simulink library "syntheticFlowGenerator"  (R2020a)
settings: Solver=VariableStepAuto  StartTime=0.0  StopTime=10.0  RelTol=1e-3
libraries: simulink x1
settings Model: Creator=Ayaz  LastModifiedBy=Ayaz

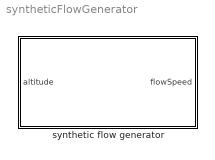
== system syntheticFlowGenerator ==
  synthetic flow generator : Subsystem  mask{hTau='exponential', timeScale=22*60, powerLawParams=[3.77 0.14], tSamp=1*60, finalTime=3*60*60, stdDev=0.5, minFlow=5, rngSeed=1, altScale=200, covAmp=1, zDiscrete=100:100:1000}
      mask prompts: hTau "Temporal kernel"; timeScale "Time scale [s]"; powerLawParams "Power law parameters, mX = a*z^b"; tSamp "Sampling time [s]"; finalTime "Timeseries end time [s]"; stdDev "Flow standard deviation [m/s]"; minFlow "Minimum flow speed [m/s]"; rngSeed "RNG seed"; altScale "Altitude length scale [m]"; covAmp "Altutude covariance amplitude [-]"; zDiscrete "Discretized altitudes [m]"
      mask init:
      | [synFlowSpeed,synFlowAlts] = generateSyntheticFlowData(hTau,...
      |     zDiscrete,finalTime,tSamp,altScale,covAmp,timeScale,...
      |     stdDev,powerLawParams,minFlow,rngSeed);
      mask DialogControl ParameterGroupVar Prompt: Temporal and mean parameters
      mask DialogControl Container3 Prompt: Synthetic flow parameters
      mask DialogControl Container4 Prompt: Altitude parameters

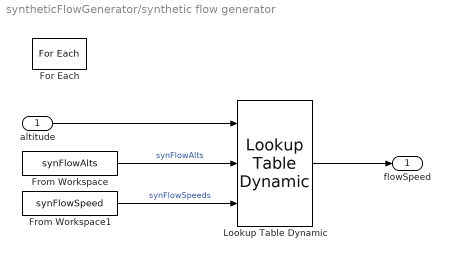
== system syntheticFlowGenerator/synthetic flow generator ==
  altitude : Inport  Partition=on  PartitionDimension=1  PartitionWidth=1  PartitionOffset=0
  For Each : ForEach  DisableCoverage=on
  From Workspace : FromWorkspace  VariableName=synFlowAlts
  From Workspace1 : FromWorkspace  VariableName=synFlowSpeed
  Lookup Table Dynamic : simulink/Lookup Tables/Lookup Table Dynamic  LookUpMeth=Interpolation-Use End Values  OutDataType=fixdt('double')  OutScaling=2^-10  OutputDataTypeScalingMode=Specify via dialog  OutDataTypeStr=double  DoSatur=off
  flowSpeed : Outport  ConcatenationDimension=1
  wires:
  altitude/1 -> Lookup Table Dynamic/1
  From Workspace/1 -> Lookup Table Dynamic/2  "synFlowAlts"
  From Workspace1/1 -> Lookup Table Dynamic/3  "synFlowSpeeds"
  Lookup Table Dynamic/1 -> flowSpeed/1
